simulink model "BiCopter_HOCBF_Landing"  (R2024a)
settings: Solver=ode4  StartTime=0.0  StopTime=100  FixedStep=0.005  RelTol=1e-3
values from neighbouring files (symbols this model uses):
  k = lqr(A,B,Q,R)    [K_Mat.m]
libraries: simulink_extras x6, shared6dof x1, fuzblock x1
settings Model: Creator=moham  LastModifiedBy=sepehrmahfar
settings OptimizationCC: ReuseModelBlockBuffer=off
settings RTWCC: GPUComputeCapability=3.5

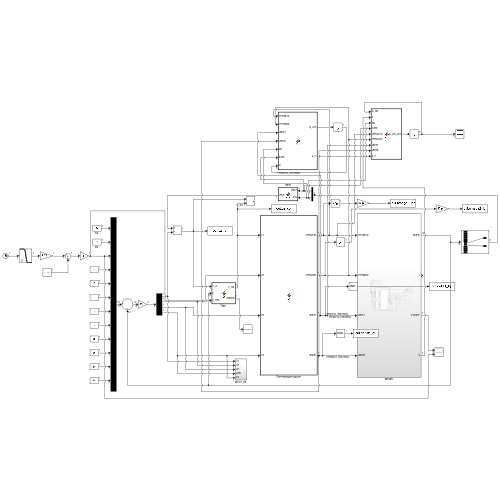
[thumbnail: Simulink's stored preview of the top-level diagram]
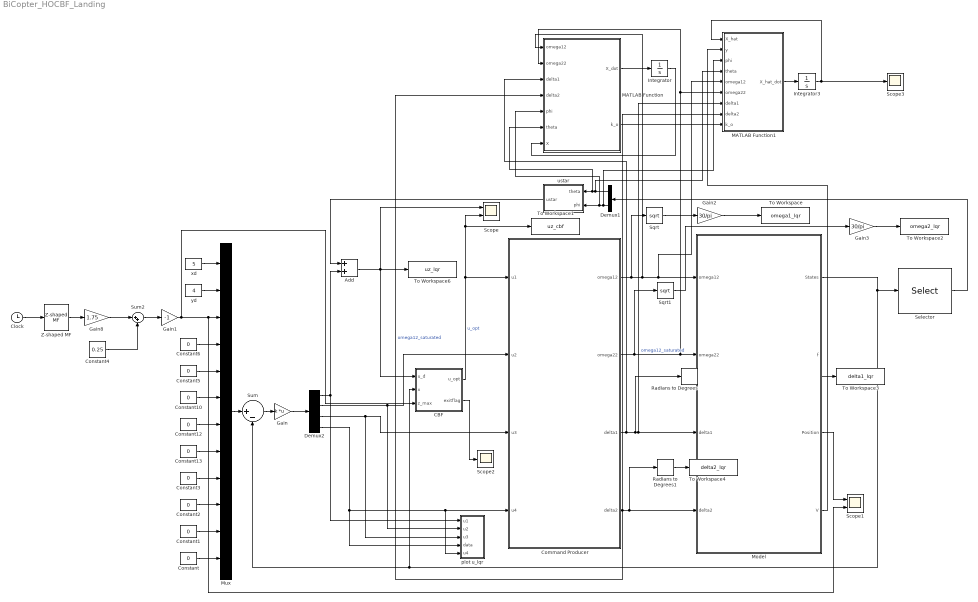
== system BiCopter_HOCBF_Landing ==
  Add : Sum
  CBF : MATLAB Function  TreatAsAtomicUnit=on
  Clock : Clock
  Command Producer : MATLAB Function  TreatAsAtomicUnit=on
  Constant{,1..3,5..6,10,12..13} (9 alike) : Constant  Value=0
  Constant4 : Constant  Value=0.25
  Demux1 : Demux  Outputs=2
  Demux2 : Demux
  Gain : Gain  Gain=k  Multiplication=Matrix(K*u)
  Gain1 : Gain  Gain=-1
  Gain2 : Gain  Gain=30/pi
  Gain3 : Gain  Gain=30/pi
  Gain8 : Gain  Gain=1.75
  Integrator : Integrator  InitialCondition=[0 ; 0; 0; 0; 0; 0]
  Integrator3 : Integrator  InitialCondition=[0; 0; 0; 0; 0; 0]
  MATLAB Function : MATLAB Function  TreatAsAtomicUnit=on
  MATLAB Function1 : MATLAB Function  TreatAsAtomicUnit=on
  Model : Subsystem
  Mux : Mux  Inputs=12
  Radians to Degrees : simulink_extras/Transformations/Radians to Degrees
  Radians to Degrees1 : simulink_extras/Transformations/Radians to Degrees
  Scope : Scope  NumInputPorts=2
  Scope1 : Scope  NumInputPorts=2
  Scope2 : Scope
  Scope3 : Scope
  Selector : Selector  InputPortWidth=12  IndexOptions=Index vector (dialog)  Indices=[7 8]  OutputSizes=1
  Sqrt : Sqrt
  Sqrt1 : Sqrt
  Sum : Sum  Inputs=|+-
  Sum2 : Sum  Inputs=|++
  To Workspace : ToWorkspace  VariableName=omega1_lqr  SaveFormat=Timeseries  SampleTime=-1
  To Workspace1 : ToWorkspace  VariableName=uz_cbf  SampleTime=-1
      settings: Save2DSignal=2-D array (concatenate along first dimension)
  To Workspace2 : ToWorkspace  VariableName=omega2_lqr  SaveFormat=Timeseries  SampleTime=-1
  To Workspace3 : ToWorkspace  VariableName=delta1_lqr  SaveFormat=Timeseries  SampleTime=-1
  To Workspace4 : ToWorkspace  VariableName=delta2_lqr  SaveFormat=Timeseries  SampleTime=-1
  To Workspace6 : ToWorkspace  VariableName=uz_lqr  SampleTime=-1
      settings: Save2DSignal=2-D array (concatenate along first dimension)
  Z-shaped MF : fuzblock/Membership  Functions/Z-shaped MF  a=10  b=15
  plot u_lqr : Subsystem
  ustar : MATLAB Function  TreatAsAtomicUnit=on
  xd : Constant  Value=5
  yd : Constant  Value=4
  wires:
  Constant/1 -> Mux/12
  Model/1(States) -> Selector/1, CBF/2(x), Sum/2
  Mux/1 -> Sum/1
  Constant1/1 -> Mux/11
  Constant2/1 -> Mux/10
  Constant6/1 -> Mux/4
  Constant5/1 -> Mux/5
  Constant10/1 -> Mux/6
  Gain1/1 -> CBF/3(z_max), Scope1/2, Mux/3
  Command Producer/1(omega12) -> Sqrt/1, MATLAB Function/1(omega12), MATLAB Function1/5(omega12), Model/1(omega12)
  Demux2/4 -> plot u_lqr/4(data), plot u_lqr/5(u4), Command Producer/4(u4)
  Demux2/3 -> plot u_lqr/3(u3), Command Producer/3(u3)
  Demux2/2 -> plot u_lqr/2(u2), Command Producer/2(u2)
  ustar/1(ustar) -> Add/1
  Constant12/1 -> Mux/7
  Constant13/1 -> Mux/8
  Sum/1 -> Gain/1
  CBF/1(u_opt) -> Command Producer/1(u1), Scope/2, To Workspace1/1  "u_opt"
  Gain/1 -> Demux2/1
  Demux2/1 -> plot u_lqr/1(u1), Add/2
  xd/1 -> Mux/1
  yd/1 -> Mux/2
  Selector/1 -> Demux1/1
  Demux1/2 -> MATLAB Function1/3(phi), MATLAB Function/5(phi), ustar/2(phi)
  Demux1/1 -> MATLAB Function1/4(theta), MATLAB Function/6(theta), ustar/1(theta)
  Model/3(Position) -> Scope1/1
  Constant3/1 -> Mux/9
  CBF/2(exitflag) -> Scope2/1
  Add/1 -> CBF/1(u_d), To Workspace6/1, Scope/1
  Sqrt/1 -> Gain2/1
  Command Producer/2(omega22) -> Sqrt1/1, MATLAB Function1/6(omega22), MATLAB Function/2(omega22), Model/2(omega22)
  Sqrt1/1 -> Gain3/1
  Command Producer/3(delta1) -> Radians to Degrees/1, Model/3(delta1), MATLAB Function1/7(delta1), MATLAB Function/3(delta1)  "omega12_saturated"
  Radians to Degrees/1 -> To Workspace3/1
  Command Producer/4(delta2) -> Model/4(delta2), Radians to Degrees1/1, MATLAB Function1/8(delta2), MATLAB Function/4(delta2)  "omega12_saturated"
  Radians to Degrees1/1 -> To Workspace4/1
  Gain2/1 -> To Workspace/1
  Gain3/1 -> To Workspace2/1
  Clock/1 -> Z-shaped MF/1
  Z-shaped MF/1 -> Gain8/1
  Gain8/1 -> Sum2/1
  Sum2/1 -> Gain1/1
  Constant4/1 -> Sum2/2
  Model/4(V) -> MATLAB Function1/2(y)
  MATLAB Function1/1(X_hat_dot) -> Integrator3/1
  Integrator3/1 -> MATLAB Function1/1(X_hat), Scope3/1
  MATLAB Function/1(X_dot) -> Integrator/1
  Integrator/1 -> MATLAB Function/7(X)
  MATLAB Function/2(k_o) -> MATLAB Function1/9(k_o)

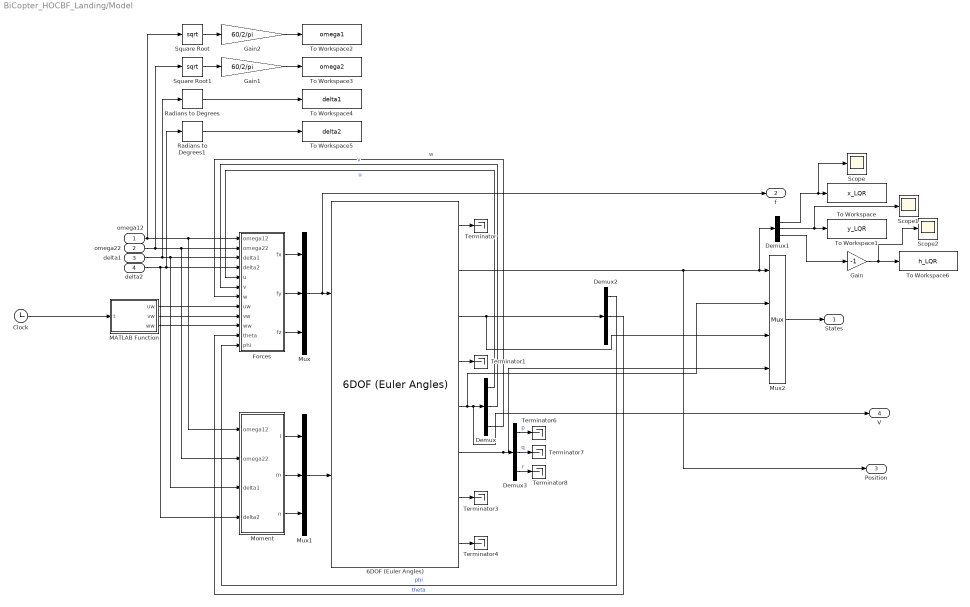
== system BiCopter_HOCBF_Landing/Model ==
  omega12 : Inport
  omega22 : Inport  Port=2
  delta1 : Inport  Port=3
  delta2 : Inport  Port=4
  6DOF (Euler Angles) : shared6dof/6DOF (Euler Angles)  units=Metric (MKS)  mtype=Fixed  rep=Euler Angles  xme_0=[0 0 -5]  Vm_0=[0 0 0]  eul_0=[0 0 0]  pm_0=[0 0 0]  mass_0=0.296  mass_e=0.5  mass_f=2.0  inertia=[0.0049, 0, -0.003675; 0, 0.0049, 0; -0.003675, 0, 0.0088]  inertia_e=eye(3)  inertia_f=2*eye(3)  k_quat=1.0  vre_flag=on  abi_flag=off  aMode=0  xme_statename=''  Vm_statename=''  eul_statename=''  quat_statename=''  pm_statename=''  mass_statename=''
  Clock : Clock
  Demux{,1..3} (4 alike) : Demux  Outputs=3
  Forces : MATLAB Function  TreatAsAtomicUnit=on
  Gain : Gain  Gain=-1
  Gain1 : Gain  Gain=60/2/pi
  Gain2 : Gain  Gain=60/2/pi
  MATLAB Function : MATLAB Function  TreatAsAtomicUnit=on
  Moment : MATLAB Function  TreatAsAtomicUnit=on
  Mux : Mux  Inputs=3
  Mux1 : Mux  Inputs=3
  Mux2 : Mux
  Radians to Degrees : simulink_extras/Transformations/Radians to Degrees
  Radians to Degrees1 : simulink_extras/Transformations/Radians to Degrees
  Scope : Scope
  Scope1 : Scope
  Scope2 : Scope
  Square Root : Sqrt
  Square Root1 : Sqrt
  Terminator{,1,3..4,6..8} (7 alike) : Terminator
  To Workspace : ToWorkspace  VariableName=x_LQR  SampleTime=-1
      settings: Save2DSignal=2-D array (concatenate along first dimension)
  To Workspace1 : ToWorkspace  VariableName=y_LQR  SampleTime=-1
      settings: Save2DSignal=2-D array (concatenate along first dimension)
  To Workspace2 : ToWorkspace  VariableName=omega1  SampleTime=-1
      settings: Save2DSignal=2-D array (concatenate along first dimension)
  To Workspace3 : ToWorkspace  VariableName=omega2  SampleTime=-1
      settings: Save2DSignal=2-D array (concatenate along first dimension)
  To Workspace4 : ToWorkspace  VariableName=delta1  SampleTime=-1
      settings: Save2DSignal=2-D array (concatenate along first dimension)
  To Workspace5 : ToWorkspace  VariableName=delta2  SampleTime=-1
      settings: Save2DSignal=2-D array (concatenate along first dimension)
  To Workspace6 : ToWorkspace  VariableName=h_LQR  SampleTime=-1
      settings: Save2DSignal=2-D array (concatenate along first dimension)
  States : Outport
  f : Outport  Port=2
  Position : Outport  Port=3
  V : Outport  Port=4
  wires:
  Moment/1(l) -> Mux1/1
  delta1/1 -> Moment/3(delta1), Forces/3(delta1), Radians to Degrees/1
  6DOF (Euler Angles)/5 -> Mux2/2, V/1, Demux/1
  Demux2/2 -> Forces/11(theta)  "theta"
  Mux/1 -> f/1, 6DOF (Euler Angles)/1
  6DOF (Euler Angles)/2 -> Position/1, Demux1/1, Mux2/1
  Forces/1(fx) -> Mux/1
  Forces/2(fy) -> Mux/2
  Mux1/1 -> 6DOF (Euler Angles)/2
  6DOF (Euler Angles)/4 -> Terminator1/1
  Demux/1 -> Forces/5(u)  "u"
  Clock/1 -> MATLAB Function/1(t)
  Demux2/1 -> Forces/12(phi)  "phi"
  Demux/2 -> Forces/6(v)  "v"
  omega12/1 -> Moment/1(omega12), Forces/1(omega12), Square Root/1
  6DOF (Euler Angles)/8 -> Terminator4/1
  6DOF (Euler Angles)/1 -> Terminator/1
  Moment/3(n) -> Mux1/3
  6DOF (Euler Angles)/7 -> Terminator3/1
  Moment/2(m) -> Mux1/2
  Forces/3(fz) -> Mux/3
  Demux/3 -> Forces/7(w)  "w"
  6DOF (Euler Angles)/3 -> Mux2/3, Demux2/1
  6DOF (Euler Angles)/6 -> Mux2/4, Demux3/1
  omega22/1 -> Moment/2(omega22), Forces/2(omega22), Square Root1/1
  delta2/1 -> Radians to Degrees1/1, Forces/4(delta2), Moment/4(delta2)
  Demux3/1 -> Terminator6/1  "p"
  Demux3/2 -> Terminator7/1  "q"
  Demux3/3 -> Terminator8/1  "r"
  Mux2/1 -> States/1
  Demux1/2 -> Scope1/1, To Workspace1/1
  Demux1/1 -> Scope/1, To Workspace/1
  Square Root/1 -> Gain2/1
  Square Root1/1 -> Gain1/1
  Radians to Degrees/1 -> To Workspace4/1
  Radians to Degrees1/1 -> To Workspace5/1
  Demux1/3 -> Gain/1
  Gain/1 -> Scope2/1, To Workspace6/1
  Gain1/1 -> To Workspace3/1
  Gain2/1 -> To Workspace2/1
  MATLAB Function/3(ww) -> Forces/10(ww)
  MATLAB Function/2(vw) -> Forces/9(vw)
  MATLAB Function/1(uw) -> Forces/8(uw)

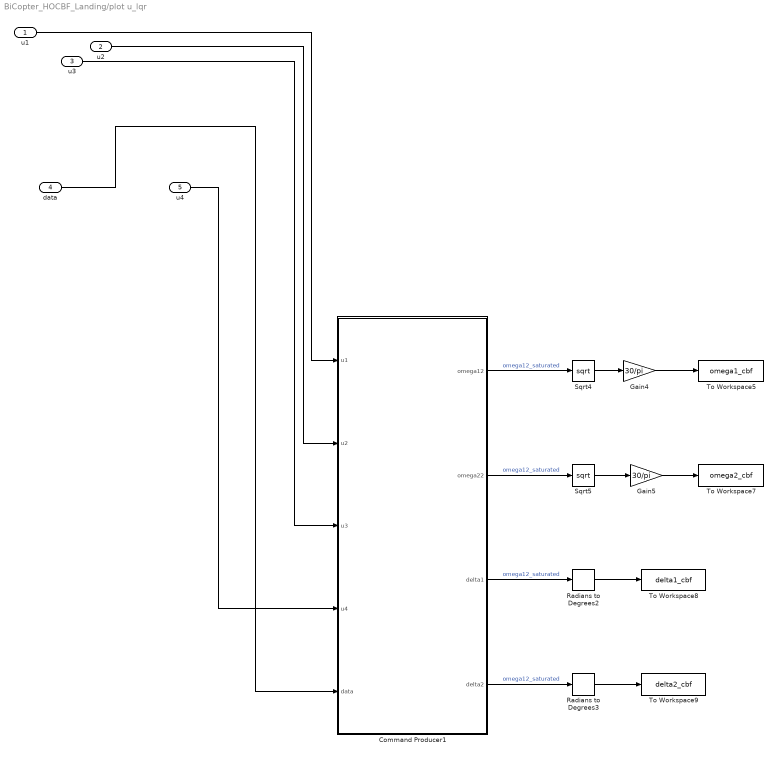
== system BiCopter_HOCBF_Landing/plot u_lqr ==
  u1 : Inport
  u2 : Inport  Port=2
  u3 : Inport  Port=3
  data : Inport  Port=4
  u4 : Inport  Port=5
  Command Producer1 : MATLAB Function  TreatAsAtomicUnit=on
  Gain4 : Gain  Gain=30/pi
  Gain5 : Gain  Gain=30/pi
  Radians to Degrees2 : simulink_extras/Transformations/Radians to Degrees
  Radians to Degrees3 : simulink_extras/Transformations/Radians to Degrees
  Sqrt4 : Sqrt
  Sqrt5 : Sqrt
  To Workspace5 : ToWorkspace  VariableName=omega1_cbf  SaveFormat=Timeseries  SampleTime=-1
  To Workspace7 : ToWorkspace  VariableName=omega2_cbf  SaveFormat=Timeseries  SampleTime=-1
  To Workspace8 : ToWorkspace  VariableName=delta1_cbf  SaveFormat=Timeseries  SampleTime=-1
  To Workspace9 : ToWorkspace  VariableName=delta2_cbf  SaveFormat=Timeseries  SampleTime=-1
  wires:
  data/1 -> Command Producer1/5(data)
  Radians to Degrees2/1 -> To Workspace8/1
  Radians to Degrees3/1 -> To Workspace9/1
  Command Producer1/2(omega22) -> Sqrt5/1  "omega12_saturated"
  Gain5/1 -> To Workspace7/1
  Command Producer1/3(delta1) -> Radians to Degrees2/1  "omega12_saturated"
  Sqrt4/1 -> Gain4/1
  u3/1 -> Command Producer1/3(u3)
  u2/1 -> Command Producer1/2(u2)
  u4/1 -> Command Producer1/4(u4)
  Command Producer1/1(omega12) -> Sqrt4/1  "omega12_saturated"
  Sqrt5/1 -> Gain5/1
  u1/1 -> Command Producer1/1(u1)
  Gain4/1 -> To Workspace5/1
  Command Producer1/4(delta2) -> Radians to Degrees3/1  "omega12_saturated"

== matlab function BiCopter_HOCBF_Landing/MATLAB Function ==
  data: omega12 input; omega22 input; delta1 input; delta2 input; phi input; theta input; X input; X_dot output; k_o output
function [X_dot, k_o] = fcn(omega12, omega22, delta1, delta2, phi, theta, X)

u = X(1);
v = X(2);
w = X(3);
uw = X(4);
vw = X(5);
ww = X(6);
m = 0.296;
g = 9.81;
rho = 1.2682;
s = 0.25;
CD = 0.32;
b = 2.98e-6;
u_dot = -g*sin(theta) - 0.5/m*rho*s*CD*sqrt((u - uw)^2+(v - vw)^2+(w - ww)^2)*(u - uw) + b/m*(omega12*sin(delta1)+omega22*sin(delta2));
v_dot = g*sin(phi)*cos(theta) - 0.5/m*rho*s*CD*sqrt((u - uw)^2+(v - vw)^2+(w - ww)^2)*(v - vw);
w_dot = g*cos(phi)*cos(theta) - 0.5/m*rho*s*CD*sqrt((u - uw)^2+(v - vw)^2+(w - ww)^2)*(w - ww) - b/m*(omega12*cos(delta1)+omega22*cos(delta2));
u_w_dot = 0;
v_w_dot = 0;
w_w_dot = 0;
X_dot = [u_dot; v_dot; w_dot; u_w_dot; v_w_dot; w_w_dot];
C = [1 0 0 0 0 0;
     0 1 0 0 0 0;
     0 0 1 0 0 0];
A = [- (6341*sqrt((u - uw)^2 + (v - vw)^2 + (w - ww)^2))/37000 - (6341*(2*u - 2*uw)*(u - uw))/(74000*sqrt((u - uw)^2 + (v - vw)^2 + (w - ww)^2)), -(6341*(2*v - 2*vw)*(u - uw))/(74000*sqrt((u - uw)^2 + (v - vw)^2 + (w - ww)^2)), -(6341*(2*w - 2*ww)*(u - uw))/(74000*sqrt((u - uw)^2 + (v - vw)^2 + (w - ww)^2)), (6341*sqrt((u - uw)^2 + (v - vw)^2 + (w - ww)^2))/37000 + (6341*(2*u - 2*uw)*(u - uw))/(74000*sqrt((u - uw)^2 + (v - vw)^2 + (w - ww)^2)), (6341*(2*v - 2*vw)*(u - uw))/(74000*sqrt((u - uw)^2 + (v - vw)^2 + (w - ww)^2)), (6341*(2*w - 2*ww)*(u - uw))/(74000*sqrt((u - uw)^2 + (v - vw)^2 + (w - ww)^2)); -(6341*(2*u - 2*uw)*(v - vw))/(74000*sqrt((u - uw)^2 + (v - vw)^2 + (w - ww)^2)), - (6341*sqrt((u - uw)^2 + (v - vw)^2 + (w - ww)^2))/37000 - (6341*(2*v - 2*vw)*(v - vw))/(74000*sqrt((u - uw)^2 + (v - vw)^2 + (w - ww)^2)), -(6341*(2*w - 2*ww)*(v - vw))/(74000*sqrt((u - uw)^2 + (v - vw)^2 + (w - ww)^2)), (6341*(2*u - 2*uw)*(v - vw))/(74000*sqrt((u - uw)^2 + (v - vw)^2 + (w - ww)^2)), (6341*sqrt((u - uw)^2 + (v - vw)^2 + (w - ww)^2))/37000 + (6341*(2*v - 2*vw)*(v - vw))/(74000*sqrt((u - uw)^2 + (v - vw)^2 + (w - ww)^2)), (6341*(2*w - 2*ww)*(v - vw))/(74000*sqrt((u - uw)^2 + (v - vw)^2 + (w - ww)^2)); -(6341*(2*u - 2*uw)*(w - ww))/(74000*sqrt((u - uw)^2 + (v - vw)^2 + (w - ww)^2)), -(6341*(2*v - 2*vw)*(w - ww))/(74000*sqrt((u - uw)^2 + (v - vw)^2 + (w - ww)^2)), - (6341*sqrt((u - uw)^2 + (v - vw)^2 + (w - ww)^2))/37000 - (6341*(2*w - 2*ww)*(w - ww))/(74000*sqrt((u - uw)^2 + (v - vw)^2 + (w - ww)^2)), (6341*(2*u - 2*uw)*(w - ww))/(74000*sqrt((u - uw)^2 + (v - vw)^2 + (w - ww)^2)), (6341*(2*v - 2*vw)*(w - ww))/(74000*sqrt((u - uw)^2 + (v - vw)^2 + (w - ww)^2)), (6341*sqrt((u - uw)^2 + (v - vw)^2 + (w - ww)^2))/37000 + (6341*(2*w - 2*ww)*(w - ww))/(74000*sqrt((u - uw)^2 + (v - vw)^2 + (w - ww)^2)); 0, 0, 0, 0, 0, 0; 0, 0, 0, 0, 0, 0; 0, 0, 0, 0, 0, 0];

P = [-5 -6 -7 -8 -9 -10]; 
k_o_t = place(A',C',P);
k_o = k_o_t';

== matlab function BiCopter_HOCBF_Landing/MATLAB Function1 ==
  data: X_hat input; X_hat_dot output; y input; phi input; theta input; omega12 input; omega22 input; delta1 input; delta2 input; k_o input
function X_hat_dot = fcn(X_hat,y, phi, theta, omega12, omega22, delta1, delta2, k_o)
m = 0.296;
g = 9.81;
rho = 1.2682;
s = 0.25;
CD = 0.32;
b = 2.98e-6;
u_hat = X_hat(1);
v_hat = X_hat(2);
w_hat = X_hat(3);
uw_hat = X_hat(4);
vw_hat = X_hat(5);
ww_hat = X_hat(6);
u_dot_hat = -g*sin(theta) - 0.5/m*rho*s*CD*sqrt((u_hat - uw_hat)^2+(v_hat - vw_hat)^2+(w_hat - ww_hat)^2)*(u_hat - uw_hat) + b/m*(omega12*sin(delta1)+omega22*sin(delta2));
v_dot_hat = g*sin(phi)*cos(theta) - 0.5/m*rho*s*CD*sqrt((u_dot_hat - uw_hat)^2+(v_hat - vw_hat)^2+(w_hat - ww_hat)^2)*(v_hat - vw_hat);
w_dot_hat = g*cos(phi)*cos(theta) - 0.5/m*rho*s*CD*sqrt((u_hat - uw_hat)^2+(v_hat - vw_hat)^2+(w_hat - ww_hat)^2)*(w_hat - ww_hat) - b/m*(omega12*cos(delta1)+omega22*cos(delta2));
u_w_dot_hat = 0;
v_w_dot_hat = 0;
w_w_dot_hat = 0;
fgu_hat = [u_dot_hat; v_dot_hat; w_dot_hat; u_w_dot_hat; v_w_dot_hat; w_w_dot_hat];

C = [1 0 0 0 0 0;
     0 1 0 0 0 0;
     0 0 1 0 0 0];
%%
k_o = 10*eye(6,3);
y_hat = C*X_hat;
X_hat_dot = fgu_hat + k_o*(y-y_hat);
end

== matlab function BiCopter_HOCBF_Landing/Model/Moment ==
  data: omega12 input; omega22 input; delta1 input; delta2 input; l output; m output; n output
function [l, m, n] = fcn(omega12, omega22, delta1, delta2)
a = 0.225;
h = 0.0225;
b = 2.98e-6;
d = 1.14e-7;
l = a*b*(omega12*cos(delta1)-omega22*cos(delta2)) + d*(-omega12*sin(delta1)+omega22*sin(delta2));
m = -b*h*(omega12*sin(delta1)+omega22*sin(delta2));
n = a*b*(omega12*sin(delta1)-omega22*sin(delta2)) + d*(omega12*cos(delta1)-omega22*cos(delta2));

== matlab function BiCopter_HOCBF_Landing/Model/Forces ==
  data: omega12 input; omega22 input; delta1 input; delta2 input; u input; fx output; v input; w input; uw input; vw input; ww input; theta input; phi input; fy output; fz output
function [fx, fy, fz] = fcn(omega12, omega22, delta1, delta2, u, v, w, uw, vw, ww, theta, phi)
ua = u - uw;
va = v - vw;
wa = w - ww;
m = 0.296;
g = 9.81;
rho = 1.2682;
s = 0.25;
CD = 0.32;
b = 2.98e-6;
fx = -m*g*sin(theta) - 0.5*rho*s*CD*sqrt(ua^2+va^2+wa^2)*ua + b*(omega12*sin(delta1)+omega22*sin(delta2));
fy = m*g*sin(phi)*cos(theta) - 0.5*rho*s*CD*sqrt(ua^2+va^2+wa^2)*va;
fz = m*g*cos(phi)*cos(theta) - 0.5*rho*s*CD*sqrt(ua^2+va^2+wa^2)*wa - b*(omega12*cos(delta1)+omega22*cos(delta2));

== matlab function BiCopter_HOCBF_Landing/Command Producer ==
  data: u1 input; omega12 output; omega22 output; delta1 output; delta2 output; u2 input; u3 input; u4 input
function [omega12, omega22, delta1, delta2] = fcn(u1, u2, u3, u4)
delta1 = atan2((u3+u4), (u1+u2));
delta2 = atan2((u3-u4), (u1-u2));
omega12 = 0.5 * (u1+u2) / cos(delta1);
omega22 = 0.5 * (u1-u2) / cos(delta2);
% a = 0.225;
% h = 0.0225;
% b = 2.98e-6;
% d = 1.14e-7;
% delta1 = atan2(b*h*(d*u2-b*a*u4) + ((d^2)+((b^2)*(a^2))*u3), b*h*(d*u4+b*a*u2) - h*(d^2)+((b^2)*(a^2))*u1);
% delta2 = atan2(b*h*(d*u2-b*a*u4) - ((d^2)+((b^2)*(a^2))*u3), b*h*(d*u4+b*a*u2) + h*(d^2)+((b^2)*(a^2))*u1);
% omega12 = ((b*h*(d*u2-b*a*u4) + ((d^2)+((b^2)*(a^2))*u3))^2) + (h^2)*((b*(d*u4 + b*a*u2) - ((d^2)+(b^2)*(a^2))*u1)^2) / (2*b*h*((d^2)+(b^2)*(a^2)));
% omega22 = ((b*h*(d*u2-b*a*u4) - ((d^2)+((b^2)*(a^2))*u3))^2) + (h^2)*((b*(d*u4 + b*a*u2) + ((d^2)+(b^2)*(a^2))*u1)^2) / (2*b*h*((d^2)+(b^2)*(a^2)));

== matlab function BiCopter_HOCBF_Landing/Model/MATLAB Function ==
  data: t input; uw output; vw output; ww output
function [uw, vw, ww] = fcn(t)
uw = 0;
vw = 0;
ww = 1;

== matlab function BiCopter_HOCBF_Landing/ustar ==
  data: theta input; phi input; ustar output
function ustar  = fcn(theta, phi)
g = 9.81;
b = 2.98e-6;
m = 0.296;
ustar = m * g / b * cos(theta) * cos(phi);

== matlab function BiCopter_HOCBF_Landing/plot u_lqr/Command Producer1 ==
  data: u1 input; omega12 output; omega22 output; delta1 output; delta2 output; u2 input; u3 input; u4 input; data input
function [omega12, omega22, delta1, delta2] = fcn(u1, u2, u3, u4, data)
delta1 = atan2((u3+u4), (u1+u2));
delta2 = atan2((u3-u4), (u1-u2));
omega12 = 0.5 * (u1+u2) / cos(delta1);
omega22 = 0.5 * (u1-u2) / cos(delta2);
% a = 0.225;
% h = 0.0225;
% b = 2.98e-6;
% d = 1.14e-7;
% delta1 = atan2(b*h*(d*u2-b*a*u4) + ((d^2)+((b^2)*(a^2))*u3), b*h*(d*u4+b*a*u2) - h*(d^2)+((b^2)*(a^2))*u1);
% delta2 = atan2(b*h*(d*u2-b*a*u4) - ((d^2)+((b^2)*(a^2))*u3), b*h*(d*u4+b*a*u2) + h*(d^2)+((b^2)*(a^2))*u1);
% omega12 = ((b*h*(d*u2-b*a*u4) + ((d^2)+((b^2)*(a^2))*u3))^2) + (h^2)*((b*(d*u4 + b*a*u2) - ((d^2)+(b^2)*(a^2))*u1)^2) / (2*b*h*((d^2)+(b^2)*(a^2)));
% omega22 = ((b*h*(d*u2-b*a*u4) - ((d^2)+((b^2)*(a^2))*u3))^2) + (h^2)*((b*(d*u4 + b*a*u2) + ((d^2)+(b^2)*(a^2))*u1)^2) / (2*b*h*((d^2)+(b^2)*(a^2)));

== matlab function BiCopter_HOCBF_Landing/CBF ==
  data: u_d input; u_opt output; x input; exitflag output; z_max input
function [u_opt, exitflag] = fcn(u_d, x, z_max)
w_w = 1;
m = 0.296;
g = 9.81;
rho = 1.2682;
s = 0.25;
b = 2.98e-6;
CD = 0.32;
alpha = 30;
beta = 11;
D = 0.01;
f_aff = g*cos(x(7))*cos(x(8)) - 0.5*rho*s*CD/m * sqrt(x(4)^2 + x(5)^2 + (x(6)-w_w)^2) * (x(6)-w_w);
g_aff = -b/m;
A = 2 *g_aff*(z_max-x(3));
b = -2*f_aff*(z_max-x(3))+2*x(6)^2-beta*2*(z_max-x(3))*x(6)+alpha*(z_max-x(3))^2-alpha*D^2;
options = optimoptions('fmincon','Display','off','Algorithm','sqp');
fun = @(u) (u - u_d )^2;
[u_opt,~,exitflag]  = fmincon(fun,u_d,A,b,[],[],[],[],[],options);


end
